simulink model "SimulinkModelforNTVBA"  (R2022a)
settings: Solver=VariableStepAuto  StartTime=0.0  StopTime=20  RelTol=1e-3
values from neighbouring files (symbols this model uses):
  c2 = 5    [DataforNTVBA.m]    (also in matlabcodeforNTnew1.m = 20; matlabcodeforNTwithMF.m = 20)
  k1 = 5    [DataforNTVBA.m]    (also in matlabcodeforNTnew1.m; matlabcodeforNTwithMF.m)
  k2 = 10    [DataforNTVBA.m]    (also in matlabcodeforNTnew1.m = 5; matlabcodeforNTwithMF.m)
  m1 = 55    [DataforNTVBA.m]    (also in matlabcodeforNTnew1.m = 6; matlabcodeforNTwithMF.m)
  m2 = 5    [DataforNTVBA.m]    (also in matlabcodeforNTnew1.m; matlabcodeforNTwithMF.m)
settings Model: Creator=91773  LastModifiedBy=URchandra
settings DebuggingCC: UnconnectedInputMsg=warning  UnconnectedOutputMsg=warning  UnconnectedLineMsg=warning
settings RTWCC: DLArmComputeVersion=19.05

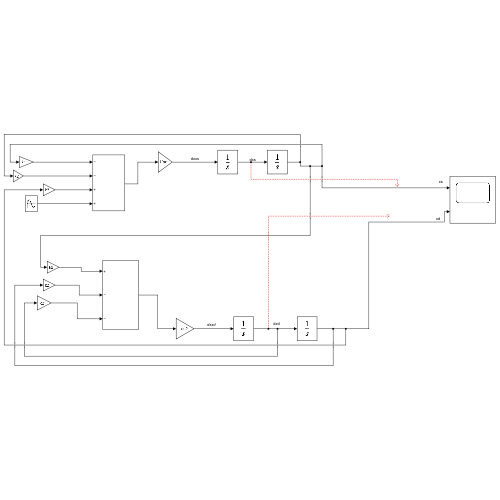
[thumbnail: Simulink's stored preview of the top-level diagram]
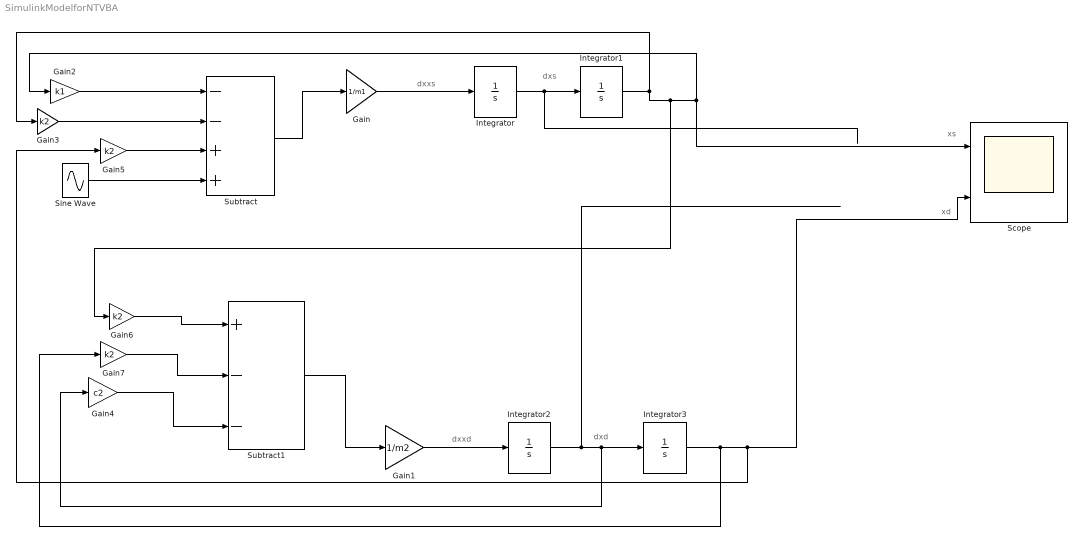
== system SimulinkModelforNTVBA ==
  note: dxxs
  note: dxd
  note: dxs
  note: dxxd
  note: xs
  note: xd
  Gain : Gain  Gain=1/m1
  Gain1 : Gain  Gain=1/m2
  Gain2 : Gain  Gain=k1
  Gain{3,5..7} (4 alike) : Gain  Gain=k2
  Gain4 : Gain  Gain=c2
  Integrator{,1..3} (4 alike) : Integrator
  Scope : Scope  NumInputPorts=2
  Sine Wave : Sin  Amplitude=20  Frequency=6  SampleTime=0
  Subtract : Sum  Inputs=--++
  Subtract1 : Sum  Inputs=+--
  wires:
  Integrator2/1 -> Gain4/1, Integrator3/1
  Gain1/1 -> Integrator2/1
  Subtract1/1 -> Gain1/1
  Integrator/1 -> Integrator1/1
  Gain/1 -> Integrator/1
  Subtract/1 -> Gain/1
  Integrator1/1 -> Gain6/1, Scope/1, Gain2/1, Gain3/1
  Gain2/1 -> Subtract/1
  Gain3/1 -> Subtract/2
  Gain5/1 -> Subtract/3
  Sine Wave/1 -> Subtract/4
  Integrator3/1 -> Gain7/1, Scope/2, Gain5/1
  Gain4/1 -> Subtract1/3
  Gain7/1 -> Subtract1/2
  Gain6/1 -> Subtract1/1
